simulink model "Week2_problem4"  (R2020b)
settings: Solver=VariableStepAuto  StartTime=0.0  StopTime=10.0  RelTol=1e-3
settings Model: DataDictionary=motor_dict.sldd  Creator=gauri  LastModifiedBy=mluser

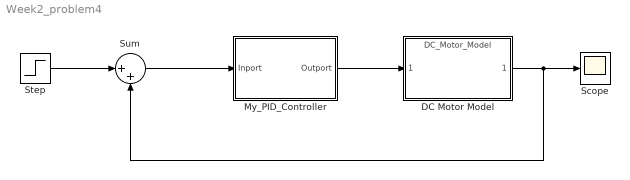
== system Week2_problem4 ==
  DC Motor Model : ModelReference  ModelNameDialog=DC_Motor_Model  UsingDefaultArgumentValue=0,0,0,0,0  SimulationMode=Normal  ModelReferenceVersion=1.20
  My_PID_Controller : Subsystem  mask{Kp=-23.0264121536819, Ki=-759.153316198618, Kd=-0.168220548295185}
      mask Display: disp('P.I.D Controller')
  Scope : Scope
  Step : Step  Time=0  After=150  SampleTime=0
  Sum : Sum  Inputs=|++
  wires:
  Step/1 -> Sum/1
  DC Motor Model/1 -> Sum/2, Scope/1
  Sum/1 -> My_PID_Controller/1(Inport)
  My_PID_Controller/1(Outport) -> DC Motor Model/1

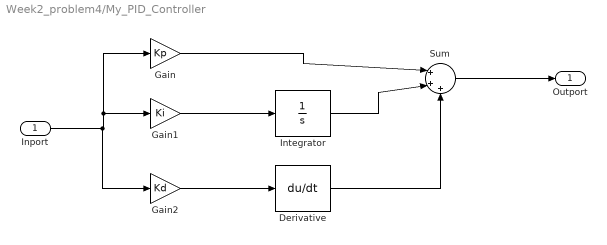
== system Week2_problem4/My_PID_Controller ==
  Inport : Inport
  Derivative : Derivative
  Gain : Gain  Gain=Kp
  Gain1 : Gain  Gain=Ki
  Gain2 : Gain  Gain=Kd
  Integrator : Integrator
  Sum : Sum  Inputs=|+++
  Outport : Outport
  wires:
  Sum/1 -> Outport/1
  Gain2/1 -> Derivative/1
  Gain/1 -> Sum/1
  Derivative/1 -> Sum/3
  Gain1/1 -> Integrator/1
  Integrator/1 -> Sum/2
  Inport/1 -> Gain2/1, Gain1/1, Gain/1
